simulink model "Main_simulation_optimised_BATTERYonly"  (R2017b)
settings: Solver=FixedStepDiscrete  StartTime=0  StopTime=20  RelTol=1e-3  EnableMultiTasking=on
PreLoadFcn:
  | Ts=2e-6;
undefined symbols (not defined in the file): DiscIntNeverNeededParam, Ion, Lithium, sigbuilder_block
libraries: powerlib x20, electricdrivelib x5, autolibshared x5, powerlib_meascontrol x3, sdolib x2, spsDrivesDcBusModel x1, spsDrivesPrivateModels x1, spsDrivesOutputSelector x1, spsDrivesSpeedControllerModel x1, simulink x1
(part 1 of 2)
Description:
  | Copyright 2008-2017 The MathWorks, Inc.
settings Model: SimulationMode=accelerator  ExtModeAutoUpdateStatusClock=off  Creator=MathWorks  LastModifiedBy=LENOVO
settings SolverCC: AlgebraicLoopSolver=LineSearch
settings DataIOCC: LimitDataPoints=on  SaveFormat=Array  SignalLoggingSaveFormat=ModelDataLogs  SaveOutput=off  SignalLogging=off  SaveTime=off  SignalLoggingName=sigsOut
settings OptimizationCC: ExpressionDepthLimit=2147483647  InitFltsAndDblsToZero=on  LifeSpan=inf
settings DebuggingCC: UnderspecifiedInitializationDetection=Classic  MergeDetectMultiDrivingBlocksExec=none  CheckExecutionContextPreStartOutputMsg=on  CheckExecutionContextRuntimeOutputMsg=on  SignalResolutionControl=TryResolveAllWithWarning  MultiTaskDSMMsg=warning  MultiTaskCondExecSysMsg=none  FcnCallInpInsideContextMsg=warning  StateNameClashWarn=warning  SFUnexpectedBacktrackingDiag=warning  SFNoUnconditionalDefaultTransitionDiag=warning  SFExecutionAtInitializationDiag=none
settings HardwareCC: ProdBitPerPointer=32  ProdBitPerSizeT=32  ProdBitPerPtrDiffT=32  ProdLargestAtomicFloat=None  ProdIntDivRoundTo=Undefined  ProdEndianess=Unspecified  ProdWordSize=32  ProdHWDeviceType=32-bit Generic  TargetUnknown=on
settings ModelReferenceCC: PropagateSignalLabelsOutOfModel=off
settings CodeAppCC: StateflowObjectComments=on
settings GRTTargetCC: TargetLangStandard=C89/C90 (ANSI)  GeneratePreprocessorConditionals=Disable all  CombineOutputUpdateFcns=off  GRTInterface=on
settings ConfigComp: CovMetricSettings=dw  CovHtmlReporting=on  CovSaveCumulativeToWorkspaceVar=on  CovSaveSingleToWorkspaceVar=on  CovExternalEMLEnable=off  CovSFcnEnable=off
settings SimscapeCC: SimscapeNormalizeSystem=off

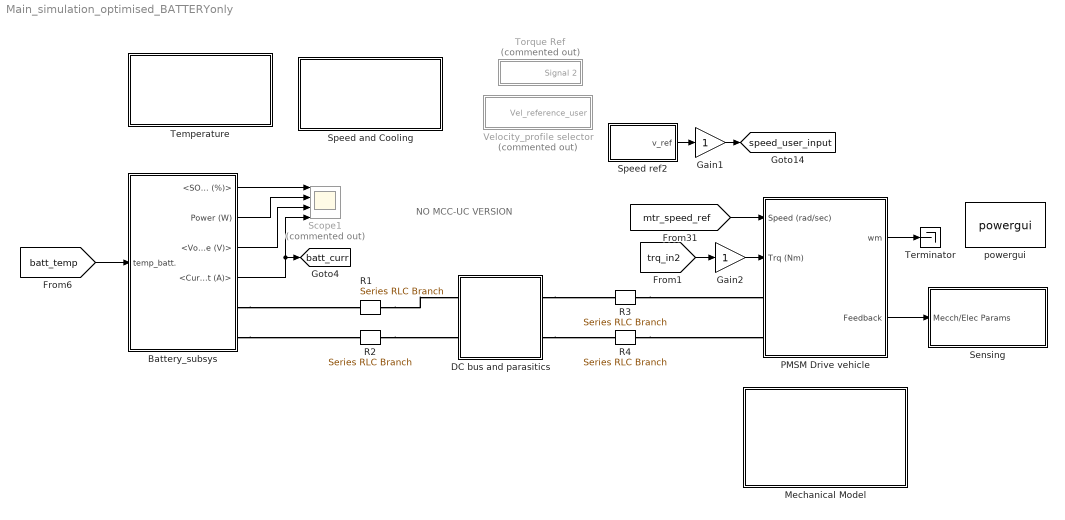
== system Main_simulation_optimised_BATTERYonly ==
  note: NO MCC-UC VERSION
  Battery_subsys : Subsystem
  DC bus and parasitics : Subsystem
  Gain1 : Gain
  Gain2 : Gain
  Mechanical Model : Subsystem
  PMSM Drive vehicle : Subsystem
  R{1..4} (4 alike) : powerlib/Elements/Series RLC Branch  LConnTagsString=__new0  RConnTagsString=__new0  BranchType=R  Resistance=0.02  Inductance=220e-6  SetiL0=off  InitialCurrent=0  Capacitance=447e-6  Setx0=off  InitialVoltage=0  Measurements=None
  Scope1 : Scope  Commented=on  NumInputPorts=4
  Sensing : Subsystem
  "Speed and Cooling " : Subsystem
  Speed ref2 : Subsystem  Tag=STV Subsys  LoadFcn=sigbuilder_block('load');  StartFcn=sigbuilder_block('start');  StopFcn=sigbuilder_block('stop');  ClipboardFcn=sigbuilder_block('clipboard');  mask(Sigbuilder block){tuvar=[0:10]}
      mask help: Simulink:masks:SigbuilderBlock_MD
      mask init:
      | if ~strcmp(get_param(bdroot(gcbh),'SimulationStatus'),'stopped') tuvar = sigbuilder_block('maskInit'); end
      settings: CopyFcn=sigbuilder_block('copy');  DeleteFcn=sigbuilder_block('delete');  ModelCloseFcn=sigbuilder_block('modelClose');  PreSaveFcn=sigbuilder_block('preSave');  PauseFcn=sigbuilder_block('pause');  ContinueFcn=sigbuilder_block('continue');  NameChangeFcn=sigbuilder_block('namechange');  OpenFcn=sigbuilder_block('open',[5.4 33 1141.2 514.8 ]);  CloseFcn=sigbuilder_block('close');
      mask Display: plot(0, 0, 100, 100,[2, 2, 32, 32, 2], [68, 8, 8, 68, 68],[32, 2], [38, 38], [32, 19, 2],[53, 60, 44], [32, 17, 17, 2],[16, 16, 31, 31]);txt = getActiveGroup(gcbh);text(2, 100, txt,'verticalAlignment', 'top');
  Temperature : Subsystem
  Terminator : Terminator
  Torque Ref : Subsystem  Tag=STV Subsys  Commented=on  LoadFcn=sigbuilder_block('load');  StartFcn=sigbuilder_block('start');  StopFcn=sigbuilder_block('stop');  ClipboardFcn=sigbuilder_block('clipboard');  mask(Sigbuilder block){tuvar=[0:10]}
      mask help: Simulink:masks:SigbuilderBlock_MD
      mask init:
      | if ~strcmp(get_param(bdroot(gcbh),'SimulationStatus'),'stopped') tuvar = sigbuilder_block('maskInit'); end
      settings: CopyFcn=sigbuilder_block('copy');  DeleteFcn=sigbuilder_block('delete');  ModelCloseFcn=sigbuilder_block('modelClose');  PreSaveFcn=sigbuilder_block('preSave');  PauseFcn=sigbuilder_block('pause');  ContinueFcn=sigbuilder_block('continue');  NameChangeFcn=sigbuilder_block('namechange');  OpenFcn=sigbuilder_block('open',[5.4 30 1141.2 522.6 ]);  CloseFcn=sigbuilder_block('close');
      mask Display: plot(0, 0, 100, 100,[2, 2, 32, 32, 2], [68, 8, 8, 68, 68],[32, 2], [38, 38], [32, 19, 2],[53, 60, 44], [32, 17, 17, 2],[16, 16, 31, 31]);txt = getActiveGroup(gcbh);text(2, 100, txt,'verticalAlignment', 'top');
  Velocity_profile selector : Subsystem  Commented=on
  powergui : powerlib/powergui  Priority=2  SimulationMode=Discrete  SampleTime=1e-6  frequency=60  Iterations=50  frequencyindice=0  Pbase=100e6  ErrMax=1e-4  UnitsV=kV  UnitsW=MW  buscounter=0  FunctionMessages=off  echomessages=off  EnableUseOfTLC=off  CurrentSourceSwitches=off  DisableSnubberDevices=off  DisableRonSwitches=off  DisableVfSwitches=off  DisplayEquations=off  SolverType=Tustin/Backward Euler (TBE)  Interpol=off  ExternalGateDelay=off  methode=off  Ts=0  x0status=blocks  SPID=off  SwTol=0  HookPort=off  RestoreLinks=warning  ResistiveCurrentMeasurement=off  Frange=[0:2:500]  Ylog=off  Xlog=on  ShowGrid=off  save=off  variable=ZData  structure=0  ZoomFFT=on  StartTime=0.0  cycles=1  DisplayStyle=1  fundamental=60  FreqAxis=off  MaxFrequency=1000  frequencyindicesteady=1  RmsSteady=1  display=off
  tag scope: batt_curr=global, speed_user_input=global
  wires:
  Speed ref2/1(v_ref) -> Gain1/1
  [trq_in2] -> Gain2/1
  Gain2/1 -> PMSM Drive vehicle/2(Trq (Nm))
  PMSM Drive vehicle/1(wm) -> Terminator/1
  PMSM Drive vehicle/2(Feedback) -> Sensing/1(Mecch/Elec Params)
  Battery_subsys/4(<Current (A)>) -> Scope1/4, [batt_curr]
  [batt_temp] -> Battery_subsys/1(temp_batt.)
  Battery_subsys/2(Power (W)) -> Scope1/2
  Battery_subsys/1(<SOC (%)>) -> Scope1/1
  Battery_subsys/3(<Voltage (V)>) -> Scope1/3
  [mtr_speed_ref] -> PMSM Drive vehicle/1(Speed (rad/sec))
  Gain1/1 -> [speed_user_input]
  connections:
  DC bus and parasitics/RConn1 -- R3/RConn1
  DC bus and parasitics/RConn2 -- R4/RConn1
  Battery_subsys/RConn1 -- R1/RConn1
  Battery_subsys/RConn2 -- R2/RConn1
  R1/LConn1 -- DC bus and parasitics/LConn1
  R2/LConn1 -- DC bus and parasitics/LConn2
  R3/LConn1 -- PMSM Drive vehicle/LConn1
  R4/LConn1 -- PMSM Drive vehicle/LConn2

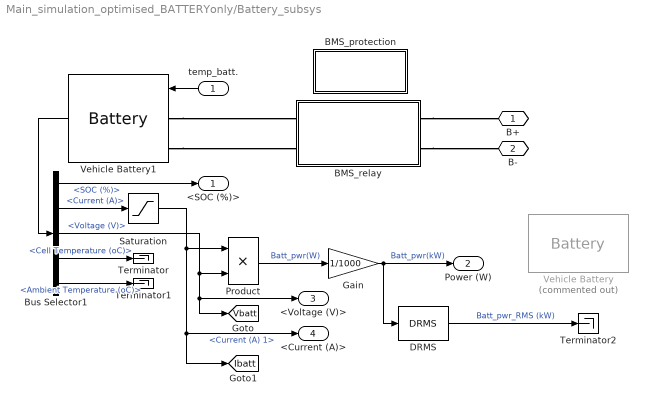
== system Main_simulation_optimised_BATTERYonly/Battery_subsys ==
  temp_batt. : Inport
  BMS_protection : Subsystem
  BMS_relay : Subsystem
  Bus Selector1 : BusSelector  OutputSignals=SOC (%),Current (A),Voltage (V),Cell Temperature (oC),Ambient Temperature (oC)
  DRMS : sdolib/RMS Blocks/DRMS  Ts=10e-6
      settings: SourceProductName=Simulink Design Optimization  SourceProductBaseCode=SO
  Gain : Gain  Gain=1/1000
  Product : Product
  Saturation : Saturate  UpperLimit=50  LowerLimit=-40
  Terminator : Terminator
  Terminator1 : Terminator
  Terminator2 : Terminator
  Vehicle Battery : electricdrivelib/Extra Sources/Battery  Commented=on  BatType=Lithium-Ion  ShowTempParam=off  ThermalPreset=no  ShowAgeParam=off  NomV=120  NomQ=66  SOC=80  Batt_Tr=30  PresetModel=off  MaxQ=66  MinV=90  FullV=130  Dis_rate=30  R=0.018182  Normal_OP=59.687  expZone="[129.6463      3.242609]"  current=[6.5 13 18 22 32.5 40]  Units=Time  Tci=20  NomT=50  T2=-15  MaxQ2=60*0.7  FullV2=117  Normal_OP2=120*0.9  expZone2="[120        50]"  Rca=0.06  ti=1000  Dp=0  Neq0=1  Tsim=1e6  Ta1=35  Qeol=60*0.85  Reol=0.013333*1.2  Char_age=[2.3478, 3]  Dis_age=[2.3478, 10]  N1=1500  N2=10500  N3=1000  N4=1400  Ta2=45  N5=950
  Vehicle Battery1 : electricdrivelib/Extra Sources/Battery  BatType=Lithium-Ion  ShowTempParam=on  ThermalPreset=no  ShowAgeParam=off  NomV=120  NomQ=66  SOC=100  Batt_Tr=0.1  PresetModel=off  MaxQ=66  MinV=90  FullV=130  Dis_rate=30  R=0.018182  Normal_OP=59.687  expZone="[129.6463      3.242609]"  current=[3.5 6.5 13 18 22 32.5 40]  Units=Time  Tci=20  NomT=50  T2=-15  MaxQ2=60*0.7  FullV2=117  Normal_OP2=120*0.9  expZone2="[120        50]"  Rca=0.5  ti=1  Dp=0  Neq0=1  Tsim=50e-6  Ta1=35  Qeol=60*0.85  Reol=0.013333*1.2  Char_age=[2.3478, 3]  Dis_age=[2.3478, 10]  N1=1500  N2=10500  N3=1000  N4=1400  Ta2=45  N5=950
  B+ : PMIOPort  Port=1  Side=Right
  B- : PMIOPort  Port=2  Side=Right
  <SOC (%)> : Outport
  Power (W) : Outport  Port=2
  <Voltage (V)> : Outport  Port=3
  <Current (A)> : Outport  Port=4
  tag scope: Ibatt=global, Vbatt=global
  wires:
  temp_batt./1 -> Vehicle Battery1/1
  Bus Selector1/2 -> Saturation/1  "<Current (A)>"
  Bus Selector1/1 -> <SOC (%)>/1  "<SOC (%)>"
  Product/1 -> Gain/1  "Batt_pwr(W)"
  Vehicle Battery1/1 -> Bus Selector1/1
  Bus Selector1/3 -> <Voltage (V)>/1, [Vbatt], Product/2  "<Voltage (V)>"
  Gain/1 -> DRMS/1, Power (W)/1  "Batt_pwr(kW)"
  Saturation/1 -> <Current (A)>/1, [Ibatt], Product/1  "<Current (A) 1>"
  Bus Selector1/4 -> Terminator/1  "<Cell Temperature (oC)>"
  Bus Selector1/5 -> Terminator1/1  "<Ambient Temperature (oC)>"
  DRMS/1 -> Terminator2/1  "Batt_pwr_RMS (kW)"
  connections:
  Vehicle Battery1/LConn1 -- BMS_relay/LConn1
  Vehicle Battery1/LConn2 -- BMS_relay/LConn2
  BMS_relay/RConn1 -- B+/RConn1
  BMS_relay/RConn2 -- B-/RConn1

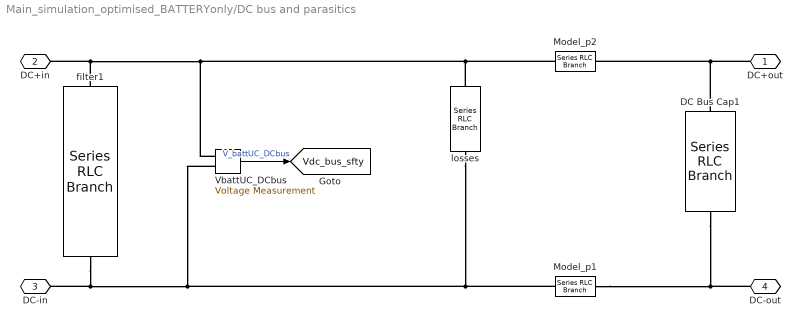
== system Main_simulation_optimised_BATTERYonly/DC bus and parasitics ==
  DC Bus Cap1 : powerlib/Elements/Series RLC Branch  LConnTagsString=__new0  RConnTagsString=__new0  BranchType=RC  Resistance=1e-2  Inductance=1e-3  SetiL0=off  InitialCurrent=0  Capacitance=400e-6  Setx0=off  InitialVoltage=0  Measurements=None
  Model_p1 : powerlib/Elements/Series RLC Branch  LConnTagsString=__new0  RConnTagsString=__new0  BranchType=RL  Resistance=0.01  Inductance=20e-6  SetiL0=off  InitialCurrent=0  Capacitance=0  Setx0=off  InitialVoltage=0  Measurements=None
  Model_p2 : powerlib/Elements/Series RLC Branch  LConnTagsString=__new0  RConnTagsString=__new0  BranchType=RL  Resistance=0.01  Inductance=20e-6  SetiL0=off  InitialCurrent=0  Capacitance=0  Setx0=off  InitialVoltage=0  Measurements=None
  VbattUC_DCbus : powerlib/Measurements/Voltage Measurement  PhasorSimulation=off  OutputType=Complex  PSBequivalent=0
  filter1 : powerlib/Elements/Series RLC Branch  LConnTagsString=__new0  RConnTagsString=__new0  BranchType=RC  Resistance=1e-3  Inductance=1e-3  SetiL0=off  InitialCurrent=0  Capacitance=1e-6  Setx0=off  InitialVoltage=0  Measurements=None
  losses : powerlib/Elements/Series RLC Branch  LConnTagsString=__new0  RConnTagsString=__new0  BranchType=R  Resistance=100e3  Inductance=1e-3  SetiL0=off  InitialCurrent=0  Capacitance=1e-6  Setx0=off  InitialVoltage=0  Measurements=None
  DC+out : PMIOPort  Port=1  Side=Right
  DC+in : PMIOPort  Port=2  Side=Left
  DC-in : PMIOPort  Port=3  Side=Left
  DC-out : PMIOPort  Port=4  Side=Right
  tag scope: Vdc_bus_sfty=global
  wires:
  VbattUC_DCbus/1 -> [Vdc_bus_sfty]  "V_battUC_DCbus"
  connections:
  DC-out/RConn1 -- Model_p1/LConn1 -- DC Bus Cap1/RConn1
  Model_p2/LConn1 -- DC+out/RConn1 -- DC Bus Cap1/LConn1
  filter1/RConn1 -- Model_p1/RConn1 -- losses/RConn1 -- VbattUC_DCbus/LConn2 -- DC-in/RConn1
  filter1/LConn1 -- Model_p2/RConn1 -- losses/LConn1 -- VbattUC_DCbus/LConn1 -- DC+in/RConn1

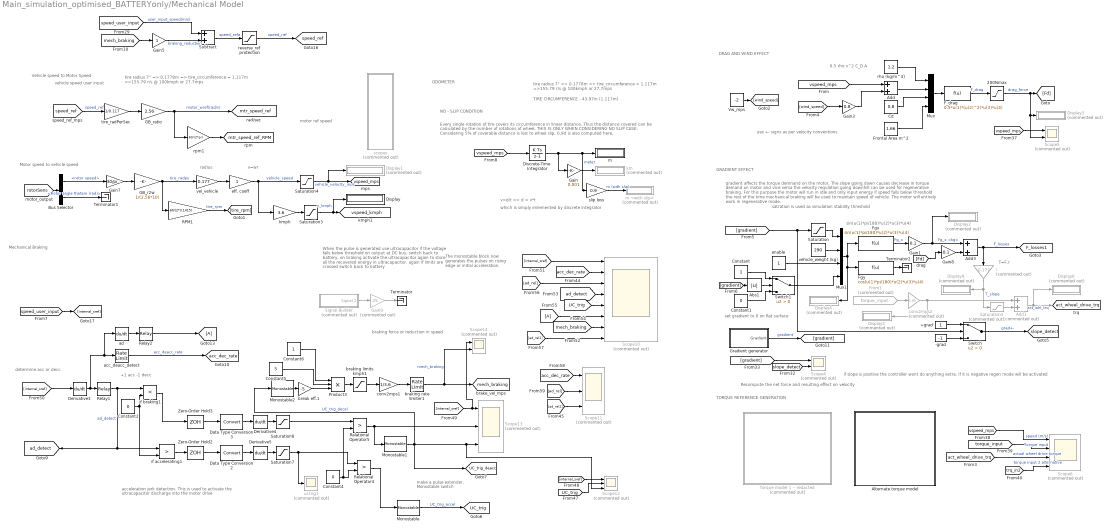
== system Main_simulation_optimised_BATTERYonly/Mechanical Model ==
  note: which is simply imlemented by discrete integrator
  note: v=d/t => d = v*t
  note: Every single rotation of tire covers its circumference in linear distance. Thus the distance covered
      | can be calculated by the number of rotations of wheel. THIS IS ONLY WHEN CONSIDERING
      | NO SLIP CASE. Considering 5% of coverable distance is lost to wheel slip, 0.9d is also computed here.
  note: TIRE CIRCUMFERENCE - 43.97in (1.117m)
  note: NO - SLIP CONDITION
  note: ODOMETER
  note: sin(u(1)*pi/180)*u(2)*u(3)*u(4)
  note: set gradient to 0 on flat surface
  note: Recompute the net force and resulting effect on velocity
  note: Vehicle speed to Motor Speed
  note: motor ref speed
  note: tire radius 7" => 0.1778m => tire_circumference = 1.117m
      | =>155.79 r/s @ 100kmph or 27.7mps
  note: vehicle speed
      | user input
  note: v=wr
  note: Motor speed to vehicle speed
  note: radius
  note: T=F.r
  note: use +- signs as per velocity conventions
  note: satration is used as simulation stability threshold
  note: gradient affects the torque demnand on the motor. The slope going down causes decrease in torque demand on motor and vice versa
      |
      | the velocity regulation going downhill can be used for regenerative braking. For this purpose the motor will run in idle and only input energy if speed falls below threshold
      | the rest of the time mechanical braking will be used to maintain speed of vehicle. The motor will entirely work in regenerative mode.
  note: if slope is positive the controller wont do anything extra. If it is negative regen mode will be activated
  note: 0.5 rho v^2 C_D A
  note: GRADIENT EFFECT
  note: DRAG AND WIND EFFECT
  note: TORQUE REFERENCE GENERATION
  note: make a pulse extender.
      | Monostable switch
  note: acceleration jerk detection. This is used to activate the ultracapacitor discharge into the motor drive
  note: When the pulse is generated use ultracapacitor
      | if the voltage falls below threshold on output
      | at DC bus, switch back to battery.
      |
      | on braking activate the ultracapacitor again to store all
      | the recovered energy in ultracapacitor. again if limits are
      | crossed switch back to battery
  note: The monostable block
      | now generates the
      | pulses on rising edge or
      | initial acceleration.
  note: Mechanical Braking
  note: braking force or reduction in speed
  note: determine acc or decc
  note: +1 acc
      |  -1 decc
  note: tire radius 7" => 0.1778m => tire_circumference = 1.117m
      | =>155.79 r/s @ 100kmph or 27.7mps
  +grad : Constant
  -grad : Constant  Value=-1
  200Nmax : Saturate  UpperLimit=200  LowerLimit=0
  Abs1 : Abs
  Add : Sum
  Add1 : Sum  Commented=on
  Add3 : Sum
  Alternate torque model : Subsystem
  Bus Selector : BusSelector  OutputSignals=rotor speed,Rotor angle thetam (rad)
  Cd : Constant  Value=0.8
  Constant : Constant
  Constant1 : Constant  Value=0
  Constant2 : Constant  Value=0
  Constant4 : Constant  Value=0
  Constant5 : Constant  Value=5
  Constant6 : Constant
  Data Type Conversion2 : DataTypeConversion
  Data Type Conversion3 : DataTypeConversion
  Derivative3 : Derivative
  Derivative4 : Derivative
  Derivative5 : Derivative
  Discrete-Time Integrator : DiscreteIntegrator  InitialConditionSetting=State (most efficient)  SampleTime=-1  ICPrevOutput=DiscIntNeverNeededParam  ICPrevScaledInput=DiscIntNeverNeededParam
  Display : Display
  Display{1..6,9} (7 alike) : Display  Commented=on
  F_drag : Fcn  Expr=0.5*u(1)*(u(2)^2)*u(3)*u(4)
  Fgx : Fcn  Expr=sin(u(1)*pi/180)*u(2)*u(3)*u(4)
  Fgy : Fcn  Expr=cos(u(1)*pi/180)*u(2)*u(3)*u(4)
  From1 : From  Commented=on  GotoTag=torque_input  TagVisibility=global
  Frontal Area m^2 : Constant  Value=1.66
  GB_r2w : Gain  Gain=1/(2.56*10)
  GB_ratio : Gain  Gain=2.56
  Gain : Gain  Gain=0.001
  Gain1 : Gain  Gain=0.1
  Gain3 : Gain  Gain=0.8
  Gain5 : Gain
  Gain7 : Gain  Gain=30/pi  SaturateOnIntegerOverflow=on  OutDataTypeStr=Inherit: Same as input  ParamDataTypeStr=Inherit: Same as input
  Gain8 : Gain  Gain=0.1
  Gain9 : Gain  Commented=on  Gain=25
  Gradient generator : Subsystem  Tag=STV Subsys  LoadFcn=sigbuilder_block('load');  StartFcn=sigbuilder_block('start');  StopFcn=sigbuilder_block('stop');  ClipboardFcn=sigbuilder_block('clipboard');  mask(Sigbuilder block){tuvar=[0:10]}
      mask help: Simulink:masks:SigbuilderBlock_MD
      mask init:
      | if ~strcmp(get_param(bdroot(gcbh),'SimulationStatus'),'stopped') tuvar = sigbuilder_block('maskInit'); end
      settings: CopyFcn=sigbuilder_block('copy');  DeleteFcn=sigbuilder_block('delete');  ModelCloseFcn=sigbuilder_block('modelClose');  PreSaveFcn=sigbuilder_block('preSave');  PauseFcn=sigbuilder_block('pause');  ContinueFcn=sigbuilder_block('continue');  NameChangeFcn=sigbuilder_block('namechange');  OpenFcn=sigbuilder_block('open',[0 30 1152 561.6 ]);  CloseFcn=sigbuilder_block('close');
      mask Display: plot(0, 0, 100, 100,[2, 2, 32, 32, 2], [68, 8, 8, 68, 68],[32, 2], [38, 38], [32, 19, 2],[53, 60, 44], [32, 17, 17, 2],[16, 16, 31, 31]);txt = getActiveGroup(gcbh);text(2, 100, txt,'verticalAlignment', 'top');
  Monostable : powerlib_meascontrol/Logic/Monostable  EdgeDetect=Rising  PulseDuration=0.4  ic=0  Ts=0
      settings: SourceProductName=Simscape Power Systems  SourceProductBaseCode=PS
  Monostable1 : powerlib_meascontrol/Logic/Monostable  EdgeDetect=Rising  PulseDuration=0.15  ic=0  Ts=0
      settings: SourceProductName=Simscape Power Systems  SourceProductBaseCode=PS
  Monostable2 : powerlib_meascontrol/Logic/Monostable  EdgeDetect=Rising  PulseDuration=0.45  ic=0  Ts=0
      settings: SourceProductName=Simscape Power Systems  SourceProductBaseCode=PS
  Mux : Mux
  Mux1 : Mux
  Product3 : Product  Inputs=3
  RPM1 : Gain  Gain=60/(2*3.1415)
  Relational Operator4 : RelationalOperator  Operator=>  OutDataTypeStr=boolean  RndMeth=Simplest
  Relational Operator5 : RelationalOperator  Operator=>  OutDataTypeStr=boolean  RndMeth=Simplest
  Relay1 : Relay  OffOutputValue=-1
  Relay2 : Relay  OffOutputValue=-1
  Saturation : Saturate  UpperLimit=10  LowerLimit=-10
  Saturation3 : Saturate  UpperLimit=108  LowerLimit=0
  Saturation4 : Saturate  UpperLimit=30  LowerLimit=0
  Saturation5 : Saturate  Commented=on  UpperLimit=25  LowerLimit=-25
  Saturation7 : Saturate  UpperLimit=10  LowerLimit=-10
  Saturation8 : Saturate  UpperLimit=10  LowerLimit=-10
  Scope10 : Scope  Commented=on  NumInputPorts=8
  Scope11 : Scope  Commented=on  NumInputPorts=3
  Scope12 : Scope  Commented=on  NumInputPorts=3
  Scope13 : Scope  Commented=on  NumInputPorts=3
  Scope14 : Scope  Commented=on  NumInputPorts=2
  Scope4 : Scope  Commented=on  NumInputPorts=2
  Scope5 : Scope  Commented=on  NumInputPorts=2
  Scope6 : Scope  Commented=on  NumInputPorts=4
  Signal Builder : Subsystem  Tag=STV Subsys  Commented=on  LoadFcn=sigbuilder_block('load');  StartFcn=sigbuilder_block('start');  StopFcn=sigbuilder_block('stop');  ClipboardFcn=sigbuilder_block('clipboard');  mask(Sigbuilder block){tuvar=[0:10]}
      mask help: Simulink:masks:SigbuilderBlock_MD
      mask init:
      | if ~strcmp(get_param(bdroot(gcbh),'SimulationStatus'),'stopped') tuvar = sigbuilder_block('maskInit'); end
      settings: CopyFcn=sigbuilder_block('copy');  DeleteFcn=sigbuilder_block('delete');  ModelCloseFcn=sigbuilder_block('modelClose');  PreSaveFcn=sigbuilder_block('preSave');  PauseFcn=sigbuilder_block('pause');  ContinueFcn=sigbuilder_block('continue');  NameChangeFcn=sigbuilder_block('namechange');  OpenFcn=sigbuilder_block('open',[5.4 30 1141.2 522.6 ]);  CloseFcn=sigbuilder_block('close');
      mask Display: plot(0, 0, 100, 100,[2, 2, 32, 32, 2], [68, 8, 8, 68, 68],[32, 2], [38, 38], [32, 19, 2],[53, 60, 44], [32, 17, 17, 2],[16, 16, 31, 31]);txt = getActiveGroup(gcbh);text(2, 100, txt,'verticalAlignment', 'top');
  Subtract : Sum
  Switch : Switch  Criteria=u2 > Threshold
  Switch1 : Switch  Criteria=u2 > Threshold
  Terminator : Terminator
  Terminator1 : Terminator
  Terminator2 : Terminator
  "Torque model 1 -- redacted" : Subsystem  Commented=on
  Vw_mps : Constant  Value=-2
  Zero-Order Hold2 : ZeroOrderHold  SampleTime=-1
  Zero-Order Hold3 : ZeroOrderHold  SampleTime=-1
  acc_deacc_detect : RateLimiter  RisingSlewLimit=1000  FallingSlewLimit=-10e5  SampleTimeMode=inherited
  ad : Derivative
  braking limits kmph1 : Saturate  UpperLimit=0  LowerLimit=-40
  braking rate limiter1 : RateLimiter  RisingSlewLimit=10  FallingSlewLimit=-100  SampleTimeMode=inherited
  break eff.1 : Gain  Gain=-5
  conv2mps1 : Gain  Gain=1/3.6
  conv2mps2 : Gain  Commented=on  Gain=1.65
  eff. coeff : Gain
  enable : Constant
  if accelerating1 : RelationalOperator  Operator=>  OutDataTypeStr=boolean  RndMeth=Simplest
  if braking1 : RelationalOperator  Operator=<  OutDataTypeStr=boolean  RndMeth=Simplest
  km : Display  Commented=on
  kmph : Gain  Gain=3.6
  m : Display
  m <with slip> : Display  Commented=on
  r : Gain  Commented=on  Gain=0.177
  reverse_ref protection : Saturate  UpperLimit=45  LowerLimit=0
  rho (kg/m^3) : Constant  Value=1.2
  rpm1 : Gain  Gain=60/(2*pi)
  scopes : Subsystem  Commented=on
  slip loss : Gain  Gain=0.9
  tire_radPerSec : Gain  Gain=1/0.117
  uctrig1 : Scope  Commented=on
  vehicle_weight (kg) : Constant  Value=290
  vel_vehicle : Gain  Gain=0.177
  tag scope: F_losses1=global, UC_trig=global, UC_trig_deacc=global, acc_dec_rate=global, act_wheel_drive_trq=global, ad_detect=global, mech_braking=global, mtr_speed_ref=global, mtr_speed_ref_RPM=global, slope_detect=global, speed_ref=global, vspeed_kmph=global, vspeed_mps=global
  wires:
  GB_ratio/1 -> rpm1/1, [mtr_speed_ref]  "motor_wref(rad/s)"
  Bus Selector/1 -> Gain7/1  "<rotor speed>"
  Bus Selector/2 -> Terminator1/1  "<Rotor angle thetam (rad)>"
  vel_vehicle/1 -> eff. coeff/1
  RPM1/1 -> [tire_rpm]  "tire_rpm"
  kmph/1 -> Saturation3/1
  Gain3/1 -> Add/2
  Add3/1 -> [F_losses1], r/1  "F_losses"
  Saturation4/1 -> Display1/1, [vspeed_mps]  "vehicle_velocity_mps"
  GB_r2w/1 -> RPM1/1, vel_vehicle/1  "tire_radps"
  [Fd] -> Gain8/1
  [speed_ref] -> tire_radPerSec/1  "speed_ref"
  [rotorSens] -> Bus Selector/1
  eff. coeff/1 -> Saturation4/1, kmph/1  "vehicle_speed"
  Vw_mps/1 -> [wind_speed]
  r/1 -> Display9/1, Saturation5/1  "T_slope"
  F_drag/1 -> 200Nmax/1  "F_drag"
  tire_radPerSec/1 -> GB_ratio/1
  rho (kg/m^3)/1 -> Mux/1
  rpm1/1 -> [mtr_speed_ref_RPM]
  Saturation3/1 -> [vspeed_kmph], Display/1  "v_kmph"
  Mux1/1 -> Fgx/1, Display4/1, Fgy/1
  Gradient generator/1(Gradient) -> [gradient]  "gradient"
  Frontal Area m^2/1 -> Mux/4
  Fgx/1 -> Gain1/1  "Fg_x"
  -grad/1 -> Switch/3
  [vspeed_mps] -> Add/1
  Cd/1 -> Mux/3
  From1/1 -> conv2mps2/1
  Add/1 -> Mux/2
  Add1/1 -> Display6/1, [act_wheel_drive_trq]  "act_whl_trq"
  Mux/1 -> F_drag/1
  Fgy/1 -> Terminator2/1
  [wind_speed] -> Gain3/1
  Switch/1 -> [slope_detect]  "grad+-"
  [gradient] -> Switch/2, Saturation/1
  +grad/1 -> Switch/1
  vehicle_weight (kg)/1 -> Mux1/2
  Gain7/1 -> GB_r2w/1
  [speed_user_input] -> Subtract/1  "user_input_speed(m/s)"
  Subtract/1 -> reverse_ref protection/1  "speed_refa"
  [vspeed_mps] -> Scope5/1
  [trq_in2] -> Scope6/4  "torque input 2 alternative"
  [act_wheel_drive_trq] -> Scope6/3  "actual wheel drive torque"
  [vspeed_mps] -> Scope6/1  "speed (m/s)"
  Gain8/1 -> Add3/2
  200Nmax/1 -> Scope5/2, Display3/1, [Fd]  "drag_force"
  [slope_detect] -> Scope4/2
  Gain5/1 -> Subtract/2  "braking_reduction"
  conv2mps1/1 -> braking rate limiter1/1
  [internal_sref] -> Derivative3/1
  [mech_braking] -> Gain5/1
  [gradient] -> Scope4/1
  [torque_input] -> Scope6/2  "Torque input"
  ad/1 -> Relay2/1
  Derivative5/1 -> Saturation7/1
  Relational Operator4/1 -> Monostable/1
  Constant2/1 -> if accelerating1/2, if braking1/2
  [ad_detect] -> Scope10/4
  [mech_braking] -> Scope10/7
  Data Type Conversion3/1 -> Derivative4/1
  Monostable1/1 -> Scope12/3, Scope13/3, [UC_trig_deacc], Monostable2/1  "UC_trig_decel"
  [ad_rel] -> Scope10/3
  [UC_trig] -> Scope12/2
  Saturation7/1 -> uctrig1/1, Relational Operator4/1
  [internal_sref] -> Scope12/1
  acc_deacc_detect/1 -> [acc_dec_rate]  "acc_deacc_rate"
  braking rate limiter1/1 -> Scope14/2, [mech_braking]  "mech_braking"
  Data Type Conversion2/1 -> Derivative5/1
  [ad_rel] -> Scope11/2
  Relational Operator5/1 -> Monostable1/1, Scope13/2
  [ad_rel2] -> Scope10/8
  Zero-Order Hold2/1 -> Data Type Conversion2/1
  [ad_rel2] -> Scope11/3
  braking limits kmph1/1 -> conv2mps1/1
  Relay2/1 -> [A]
  Constant5/1 -> Product3/2
  Monostable2/1 -> break eff.1/1
  Zero-Order Hold3/1 -> Data Type Conversion3/1
  [acc_dec_rate] -> Scope11/1
  Gain9/1 -> Terminator/1
  [UC_trig] -> Scope10/5
  Derivative4/1 -> Saturation8/1
  Monostable/1 -> [UC_trig]  "UC_trig_accel"
  [internal_sref] -> Scope14/1, Scope13/1
  [speed_user_input] -> [internal_sref]
  if accelerating1/1 -> Zero-Order Hold2/1
  Constant4/1 -> Relational Operator5/2, Relational Operator4/2
  Saturation8/1 -> Relational Operator5/1
  Constant6/1 -> Product3/1
  Signal Builder/1(Signal 2) -> Gain9/1
  break eff.1/1 -> Product3/3
  if braking1/1 -> Zero-Order Hold3/1
  [A] -> Scope10/6
  Derivative3/1 -> ad/1, acc_deacc_detect/1, Relay1/1
  Product3/1 -> braking limits kmph1/1
  Relay1/1 -> [ad_detect], if accelerating1/1, if braking1/1  "ad_detect"
  [internal_sref] -> Scope10/1
  [acc_dec_rate] -> Scope10/2
  Saturation5/1 -> Add1/2
  conv2mps2/1 -> Display5/1, Add1/1
  Gain1/1 -> Display2/1, Add3/1  "Fg_x <kg>"
  enable/1 -> Mux1/3
  [gradient] -> Abs1/1
  Abs1/1 -> Switch1/2
  Constant/1 -> Switch1/1
  Constant1/1 -> Switch1/3
  Switch1/1 -> Mux1/4
  Saturation/1 -> Mux1/1
  reverse_ref protection/1 -> [speed_ref]  "speed_ref"
  [vspeed_mps] -> Discrete-Time Integrator/1
  Discrete-Time Integrator/1 -> Gain/1, slip loss/1, m/1  "meter"
  Gain/1 -> km/1
  slip loss/1 -> m <with slip>/1  "m (with slip)"

== system Main_simulation_optimised_BATTERYonly/PMSM Drive vehicle ==
  Speed (rad/sec) : Inport
  Trq (Nm) : Inport  Port=2
  Bus Creator : BusCreator  Inputs=3
  Bus Selector : BusSelector  OutputSignals=V bus (V)
  DC_bus overvoltage protection : Subsystem  Commented=on
  PM Synchronous Motor Drive : Subsystem  DialogController=POWERSYS.PowerSysDialog  LoadFcn=|  mask(PM Synchronous Motor Drive){Rs=0.2, Lls=8.5e-3, Lms=8.5e-3, MachineConstant=Flux linkage established by magnets (V.s), FluxCst=0.175, VoltageCst=126.966, TorqueCst=1.05, ia=0, ib=0, J=0.089, Friction=0.005, p=4, wm=0, thetam=0, Rsnb_rec=10e3, Csnb_rec=20e-9, Ron_rec=1e-3, Vf_rec=1.3, cap_bus=200e-6, Rbrake=8, fbrake=4000, activationVoltage=190, shutdownVoltage=175, sourceFrequency=60, deviceType=IGBT / Diodes, Ron_inv=1e-3, Vf_inv=0.8, Vfd_inv=0.8, Tf=1e-6, Tt=2e-6, Tf_GTO=0, Tt_GTO=0, Rsnb_inv=5000, Csnb_inv=inf, regulationType=Speed regulation, Acc=1000, Dec=-1000, kp_sc=5, ki_sc=100, fc_sc=100, Tsc=7*20e-6, Tmin=-17.8, Tmax=17.8, modulationType=Hysteresis, h=0.1, kp_Id=200, ki_Id=1000, kp_Iq=200, ki_Iq=1000, fc_bus=50, car_freq=20000, freq_max=20e3, Tvect=20e-6, baseSampleTime=2e-06, outputBusMode=Multiple output buses, busLabels=off, MechanicalLoad=Torque Tm, modelDetailLevel=Detailed, driveType=AC6, AverageValue=off}
      | if ~isempty(get_param(gcb,'UserData')) 
      |       UserDataToSimulinkMask(gcbh,get_param(gcb,'driveType'));  
      |       set_param(gcb, 'UserData',[]);
      |       set_param(gcb,'UserDataPersistent','off');
      | end 
      | if strcmp(get_param(gcb,'AverageValue'),'on')
      |     set_param(gcb,'modelDetailLevel','Average');
      | end
      mask prompts: Rs "Resistance (ohm):"; Lls "D-axis inductance (H):"; Lms "Q-axis inductance (H):"; MachineConstant "Specify:"; ia "Phase A (A):"; ib "Phase B (A):"; J "Inertia (kg.m^2):"; Friction "Friction factor (N.m.s):"; p "Pole pairs:"; wm "Speed (rad/s):"; thetam "Angle (deg):"; Rsnb_rec "Resistance (ohm):"; Csnb_rec "Capacitance (F):"; Ron_rec "On-state resistance (ohm):"; Vf_rec "Forward voltage (V):"; cap_bus "Capacitance (F):"; Rbrake "Resistance (ohm):"; fbrake "Chopper frequency (Hz):"; activationVoltage "Activation voltage (V):"; shutdownVoltage "Shutdown voltage (V):"; sourceFrequency "Source frequency (Hz):"; deviceType "Device type:"; Ron_inv "On-state resistance (ohm):"; Vf_inv "Main device:"; Vfd_inv "Diode:"; Tf "Fall time (s):"; Tt "Tail time (s):"; Tf_GTO "Fall time (s):"; Tt_GTO "Tail time (s):"; Rsnb_inv "Resistance (ohm):"; Csnb_inv "Capacitance (F):"; regulationType "Regulation type:"; Acc "Acceleration:"; Dec "Deceleration:"; kp_sc "Proportional gain:"; ki_sc "Integral gain:"; fc_sc "Speed cutoff frequency (Hz):"; Tsc "Speed controller sampling time (s):"; Tmin "Negative:"; Tmax "Positive:"; modulationType "Modulation type:"; h "Current controller hysteresis bandwidth (A):"; kp_Id "Proportional gain:"; ki_Id "Integral gain:"; kp_Iq "Proportional gain:"; ki_Iq "Integral gain:"; fc_bus "DC bus voltage sensor cutoff frequency (Hz):"; car_freq "SVM switching frequency (Hz):"; freq_max "Maximum  switching frequency (Hz):"; Tvect "Controller sampling time (s):"; baseSampleTime "Base sample time:"; outputBusMode "Output bus mode:"; busLabels "Use bus labels"; MechanicalLoad "Mechanical input:"; modelDetailLevel "Model detail level:"; driveType "Drive type:"; AverageValue "Average value model"
      mask help: Implements a classical vector control drive for permanent synchronous motors.
      mask init:
      | [X1,X1m,X2,X2m,X3,X4,Y1,Y1m,Y2,Y2m,Y3,Y4,color1,color2,INp,OUTp,machineType,baseSampleTime] = spsDrivesMaskInit(gcb,driveType,AverageValue);
      settings: OpenFcn=sps_rtmsupport('OpenFcn',gcbh)
      mask Help: helpview(psbhelp)
      mask TypeOptions MachineConstant: Flux linkage established by magnets (V.s) | Voltage Constant (V_peak L-L / krpm) | Torque Constant (N.m / A_peak)
      mask Callback MachineConstant:
      | block = gcb;
      | MC = get_param(block,'MachineConstant');
      | set_param([block,'/','Permanent Magnet Synchronous Machine'],'MachineConstant',MC);
      | set_param([block,'/','VECT'],'MachineConstant',MC);
      | switch MC
      |     case 'Flux linkage established by magnets (V.s)'
      |         set_param([block,'/','Permanent Magnet Synchronous Machine'],'Flux',get_param(block,'FluxCst'))
      |     case 'Voltage Constant (V_peak L-L / krpm)'
      |         set_param([block,'/','Permanent Magnet Synchronous Machine'],'VoltageCst',get_param(block,'VoltageCst'))
      |     case 'Torque Constant (N.m / A_peak)'
      |         set_param([block,'/','Permanent Magnet Synchronous Machine'],'TorqueCst',get_param(block,'TorqueCst'))
      | end
      mask Callback FluxCst:
      | block = gcb;
      | MC = get_param(block,'MachineConstant');
      | set_param([block,'/','Permanent Magnet Synchronous Machine'],'MachineConstant',MC);
      | set_param([block,'/','VECT'],'MachineConstant',MC);
      | switch MC
      |     case 'Flux linkage established by magnets (V.s)'
      |         set_param([block,'/','Permanent Magnet Synchronous Machine'],'Flux',get_param(block,'FluxCst'))
      |     case 'Voltage Constant (V_peak L-L / krpm)'
      |         set_param([block,'/','Permanent Magnet Synchronous Machine'],'VoltageCst',get_param(block,'VoltageCst'))
      |     case 'Torque Constant (N.m / A_peak)'
      |         set_param([block,'/','Permanent Magnet Synchronous Machine'],'TorqueCst',get_param(block,'TorqueCst'))
      | end
      mask Callback VoltageCst:
      | block = gcb;
      | MC = get_param(block,'MachineConstant');
      | set_param([block,'/','Permanent Magnet Synchronous Machine'],'MachineConstant',MC);
      | set_param([block,'/','VECT'],'MachineConstant',MC);
      | switch MC
      |     case 'Flux linkage established by magnets (V.s)'
      |         set_param([block,'/','Permanent Magnet Synchronous Machine'],'Flux',get_param(block,'FluxCst'))
      |     case 'Voltage Constant (V_peak L-L / krpm)'
      |         set_param([block,'/','Permanent Magnet Synchronous Machine'],'VoltageCst',get_param(block,'VoltageCst'))
      |     case 'Torque Constant (N.m / A_peak)'
      |         set_param([block,'/','Permanent Magnet Synchronous Machine'],'TorqueCst',get_param(block,'TorqueCst'))
      | end
      mask Callback TorqueCst:
      | block = gcb;
      | MC = get_param(block,'MachineConstant');
      | set_param([block,'/','Permanent Magnet Synchronous Machine'],'MachineConstant',MC);
      | set_param([block,'/','VECT'],'MachineConstant',MC);
      | switch MC
      |     case 'Flux linkage established by magnets (V.s)'
      |         set_param([block,'/','Permanent Magnet Synchronous Machine'],'Flux',get_param(block,'FluxCst'))
      |     case 'Voltage Constant (V_peak L-L / krpm)'
      |         set_param([block,'/','Permanent Magnet Synchronous Machine'],'VoltageCst',get_param(block,'VoltageCst'))
      |     case 'Torque Constant (N.m / A_peak)'
      |         set_param([block,'/','Permanent Magnet Synchronous Machine'],'TorqueCst',get_param(block,'TorqueCst'))
      | end
      mask TypeOptions deviceType: GTO / Diodes | MOSFET / Diodes | IGBT / Diodes
      mask Callback deviceType: set_param([gcb,'/Three-phase Inverter'],'Device',get_param(gcb,'deviceType'));
      mask TypeOptions regulationType: Speed regulation | Torque regulation
      mask Callback regulationType: set_param([gcb '/Speed Controller'],'SwK',get_param(gcb,'regulationType'));
      mask TypeOptions modulationType: Hysteresis | SVM
      mask TypeOptions outputBusMode: Multiple output buses | Single output bus
      mask TypeOptions MechanicalLoad: Torque Tm | Speed w | Mechanical rotational port
      mask TypeOptions modelDetailLevel: Detailed | Average
      mask Callback modelDetailLevel:
      | if strcmp(get_param(gcb,'modelDetailLevel'),'Average')
      |    set_param(gcb,'AverageValue','on');
      | else
      |    set_param(gcb,'AverageValue','off');
      | end
      mask TypeOptions driveType: AC6
      mask DialogControl Container7 Prompt: Permanent Magnet Synchronous Machine
      mask DialogControl Container22 Prompt: Electrical parameters
      mask DialogControl Container27 Prompt: Equivalent circuit parameters
      mask DialogControl Container21 Prompt: Flux constant
      mask DialogControl Container34 Prompt: Initial currents
      mask DialogControl Container23 Prompt: Mechanical parameters
      mask DialogControl Container36 Prompt: Initial  values
      mask DialogControl Container10 Prompt: Converters and DC bus
      mask DialogControl Container28 Prompt: Rectifier
      mask DialogControl Container26 Prompt: Snubbers
      mask DialogControl Container29 Prompt: Diodes
      mask DialogControl Container30 Prompt: DC bus
      mask DialogControl Container31 Prompt: Braking chopper
      mask DialogControl Container32 Prompt: Inverter
      mask DialogControl Container37 Prompt: Switches
      mask DialogControl Forwardvoltages Prompt: Forward voltages (V)
      mask DialogControl Turnoff Prompt: Turn-off characteristics
      mask DialogControl InvSnubbers Prompt: Snubbers
      mask DialogControl Container12 Prompt: Controller
      mask DialogControl Control5 Prompt: Schematic
      mask DialogControl Control5 Callback:
      | openfig('ac6.fig','invisible');
      | movegui(gcf,'northwest');
      | set(gcf,'Visible','on');
      mask DialogControl Container33 Prompt: Speed controller
      mask DialogControl Speedramp Prompt: Speed ramps (rpm/s)
      mask DialogControl PIregulator Prompt: PI regulator
      mask DialogControl Container43 Prompt: Torque output limits (N.m)
      mask DialogControl Container35 Prompt: Vector control
      mask DialogControl d_axiscurrentregulator Prompt: d-axis current regulator
      mask DialogControl q_axiscurrentregulator Prompt: q-axis current regulator
      mask DialogControl Container47 Prompt: Parameters file options
      mask DialogControl Control3 Prompt: Load
      mask DialogControl Control3 Callback: loadValues(gcb,get_param(gcb,'driveType'));
      mask DialogControl Control4 Prompt: Save
      mask DialogControl Control4 Callback: saveValues(gcb,get_param(gcb,'driveType'));
      mask Display:
      | patch([X1 X1m],[Y1 Y1m],color1);
      | patch(X3,Y3,color2);
      | plot([X1 X1m X2 X2m X3 X4],[Y1 Y1m Y2 Y2m Y3 Y4]);
      | text(0.5,0.3,'AC6','HorizontalAlignment','center')
      | HaveSPSMec = (strcmp(MechanicalLoad,'Torque Tm') || strcmp(MechanicalLoad,'Speed w'));
      | color('blue');
      | if (HaveSPSMec==1 && strcmp(outputBusMode,'Multiple output buses'))
      |     port_label('input',2,INp)
      |     port_label('output',4,OUTp)
      | end
      | if (HaveSPSMec==1 && strcmp(outputBusMode,'Single output bus'))
      |     port_label('input',2,INp)
      |     port_label('output',2,OUTp)
      | end
  PM Synchronous Motor Drive1 : electricdrivelib/AC drives/PM Synchronous Motor Drive  Commented=on  Rs=0.2  Lls=8.5e-3  Lms=8.5e-3  MachineConstant=Flux linkage established by magnets (V.s)  FluxCst=0.175  VoltageCst=126.966  TorqueCst=1.05  ia=0  ib=0  J=0.089  Friction=0.005  p=4  wm=0  thetam=0  Rsnb_rec=10e3  Csnb_rec=20e-9  Ron_rec=1e-3  Vf_rec=1.3  cap_bus=2000e-6  Rbrake=8  fbrake=4000  activationVoltage=320  shutdownVoltage=310  sourceFrequency=60  deviceType=IGBT / Diodes  Ron_inv=1e-3  Vf_inv=0.8  Vfd_inv=0.8  Tf=1e-6  Tt=2e-6  Tf_GTO=0  Tt_GTO=0  Rsnb_inv=5000  Csnb_inv=inf  regulationType=Speed regulation  Acc=1000  Dec=-1000  kp_sc=5  ki_sc=100  fc_sc=100  Tsc=7*20e-6  Tmin=-17.8  Tmax=17.8  modulationType=Hysteresis  h=0.1  kp_Id=200  ki_Id=1000  kp_Iq=200  ki_Iq=1000  fc_bus=50  car_freq=20000  freq_max=20e3  Tvect=20e-6  baseSampleTime=2e-06  outputBusMode=Multiple output buses  busLabels=off  MechanicalLoad=Torque Tm  modelDetailLevel=Detailed  driveType=AC6  AverageValue=off
      link override VECT: machineConstant=Flux linkage established by magnets (V.s)
      settings: SourceProductName=Simscape Power Systems  SourceProductBaseCode=PS
  + : PMIOPort  Port=1  Side=Left
  - : PMIOPort  Port=2  Side=Left
  wm : Outport
  Feedback : Outport  Port=2
  wires:
  Speed (rad/sec)/1 -> PM Synchronous Motor Drive/1(SP)
  Trq (Nm)/1 -> PM Synchronous Motor Drive/2(Tm)
  PM Synchronous Motor Drive/3(Ctrl) -> Bus Creator/3
  PM Synchronous Motor Drive/2(Conv.) -> Bus Selector/1, Bus Creator/2
  PM Synchronous Motor Drive/1(Motor) -> Bus Creator/1
  PM Synchronous Motor Drive/4(Wm) -> wm/1
  Bus Creator/1 -> Feedback/1
  Bus Selector/1 -> DC_bus overvoltage protection/1(DC_Bus_Voltage)  "<V bus (V)>"
  connections:
  PM Synchronous Motor Drive/LConn1 -- DC_bus overvoltage protection/LConn1 -- +/RConn1
  PM Synchronous Motor Drive/LConn2 -- DC_bus overvoltage protection/LConn2 -- -/RConn1

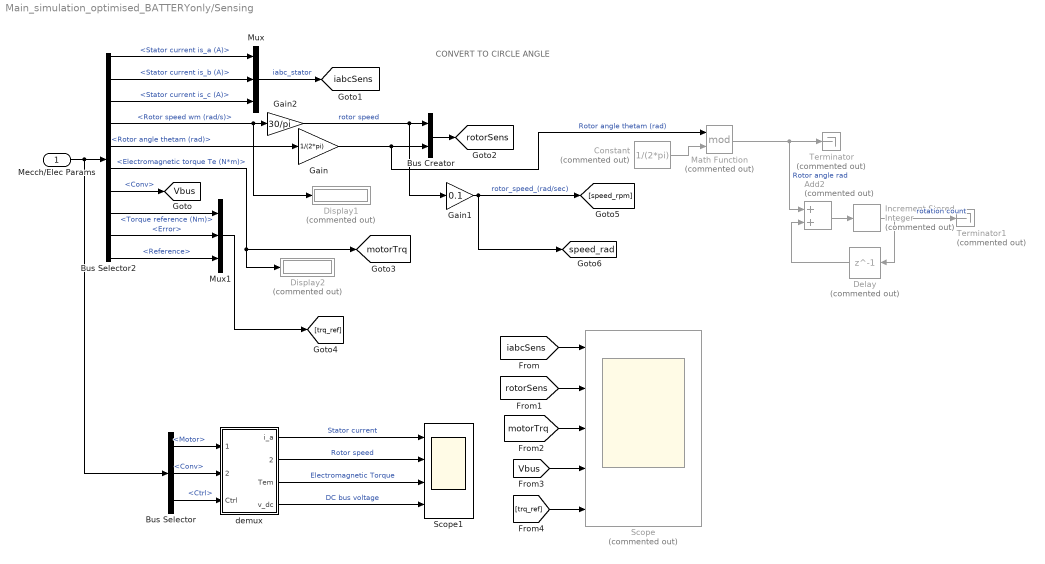
== system Main_simulation_optimised_BATTERYonly/Sensing ==
  note: CONVERT TO CIRCLE ANGLE
  Mecch/Elec Params : Inport
  Add2 : Sum  Commented=on
  Bus Creator : BusCreator  Inputs=2
  Bus Selector : BusSelector  OutputSignals=Motor,Conv,Ctrl
  Bus Selector2 : BusSelector  OutputSignals=Motor.Stator current is_a (A),Motor.Stator current is_b (A),Motor.Stator current is_c (A),Motor.Rotor speed wm (rad/s),Motor.Rotor angle thetam (rad),Motor.Electromagnetic torque Te (N*m),Conv,Ctrl.Torque reference (Nm),Ctrl.Error,Ctrl.Reference
  Constant : Constant  Commented=on  Value=1/(2*pi)
  Delay : Delay  Commented=on  DelayLength=1
  Display1 : Display  Commented=on
  Display2 : Display  Commented=on
  Gain : Gain  Gain=1/(2*pi)
  Gain1 : Gain  Gain=0.1
  Gain2 : Gain  Gain=30/pi  SaturateOnIntegerOverflow=on  OutDataTypeStr=Inherit: Same as input  ParamDataTypeStr=Inherit: Same as input
  Increment Stored Integer : simulink/Additional Math & Discrete/Additional Math: Increment - Decrement/Increment Stored Integer  Commented=on
      settings: SourceProductName=Simulink
  Math Function : Math  Commented=on  Operator=mod  SaturateOnIntegerOverflow=on
  Mux : Mux  Inputs=3
  Mux1 : Mux  Inputs=3
  Scope : Scope  Commented=on  NumInputPorts=5
  Scope1 : Scope  NumInputPorts=4
  Terminator : Terminator  Commented=on
  Terminator1 : Terminator  Commented=on
  demux : Subsystem
  tag scope: Vbus=global, iabcSens=global, motorTrq=global, rotorSens=global, speed_rad=global
  wires:
  Bus Selector2/5 -> Gain/1  "<Rotor angle thetam (rad)>"
  Mux/1 -> [iabcSens]  "iabc_stator"
  Bus Selector2/3 -> Mux/3  "<Stator current is_c (A)>"
  Mecch/Elec Params/1 -> Bus Selector/1, Bus Selector2/1
  Bus Creator/1 -> [rotorSens]
  Bus Selector2/4 -> Display1/1, Gain2/1  "<Rotor speed wm (rad/s)>"
  Bus Selector2/1 -> Mux/1  "<Stator current is_a (A)>"
  Bus Selector2/2 -> Mux/2  "<Stator current is_b (A)>"
  Bus Selector2/6 -> [motorTrq], Display2/1  "<Electromagnetic torque Te (N*m)>"
  Gain/1 -> Math Function/1, Bus Creator/2  "Rotor angle thetam (rad)"
  Bus Selector2/7 -> [Vbus]  "<Conv>"
  Bus Selector2/8 -> Mux1/1  "<Torque reference (Nm)>"
  Bus Selector2/9 -> Mux1/2  "<Error>"
  Bus Selector2/10 -> Mux1/3  "<Reference>"
  Mux1/1 -> [trq_ref]
  [iabcSens] -> Scope/1
  [rotorSens] -> Scope/2
  [motorTrq] -> Scope/3
  [Vbus] -> Scope/4
  [trq_ref] -> Scope/5
  Gain1/1 -> [speed_rad], [speed_rpm]  "rotor_speed_(rad/sec)"
  demux/2(speed) -> Scope1/2  "Rotor speed"
  demux/1(i_a) -> Scope1/1  "Stator current"
  Bus Selector/1 -> demux/1(motor)  "<Motor>"
  Bus Selector/2 -> demux/2(Conv.)  "<Conv>"
  demux/4(v_dc) -> Scope1/4  "DC bus voltage"
  demux/3(Tem) -> Scope1/3  "Electromagnetic Torque"
  Bus Selector/3 -> demux/3(Ctrl)  "<Ctrl>"
  Gain2/1 -> Gain1/1, Bus Creator/1  "rotor speed"
  Math Function/1 -> Add2/1, Terminator/1  "Rotor angle rad"
  Constant/1 -> Math Function/2
  Increment Stored Integer/1 -> Terminator1/1, Delay/1  "rotation count"
  Delay/1 -> Add2/2
  Add2/1 -> Increment Stored Integer/1

== system Main_simulation_optimised_BATTERYonly/Speed and Cooling  ==
  note: -exp(0.1*v/10)
  note: to generate speed based cooling rate
  note: not consiidering drag to keep it linear
  note: Y (kmph) = X(r/s) * 100 (kmph) / 400 (r/s)
  Gain1 : Gain  Gain=0.1/10
  Gain2 : Gain  Gain=100/400
  Math Function : Math  SaturateOnIntegerOverflow=on
  cooling_rate : Gain  Gain=-1
  tag scope: cooling_rate=global
  wires:
  Math Function/1 -> cooling_rate/1
  Gain1/1 -> Math Function/1
  [speed_rad] -> Gain2/1
  Gain2/1 -> Gain1/1
  cooling_rate/1 -> [cooling_rate]

== system Main_simulation_optimised_BATTERYonly/Speed ref2 ==
  Demux : Demux  Tag=STV Demux  Outputs=1
  FromWs : FromWorkspace  Tag=STV FromWs  VariableName=tuvar  SampleTime=0
      SigBuilderData=|
      | common.afterFinalStr = 'Extrapolate'
      | common.sampleTime = 0
      | dataSet.timeRange = [0 20]
      | dataSet.name = 'Group 1'
      | sbobj.Groups.Name = 'Group 1'
      | sbobj.Groups.Signals.Name = 'v_ref'
      | sbobj.Groups.Signals.XData = [0 1 1 2 2 2.39 2.39 3.81 5 5 6.45 6.48 6.8 7 8 8.05 9 9.1 10.2 11.4 11.58 12.5 13 13.46 14 14.26 14.48 15.04 15.2 15.4 15.5 15.64 17 18.1 18.42 18.74 19.3 19.52 20]
      | sbobj.Groups.Signals.YData = [0 5.1 0.2 11 7.5 2.4 0.6 7.1 1.2 0.4 8.7 8.1 15.3 13.2 12.9 11.3 7.1 2 2 9.26428571429 8.9 11.2014285714 16.7 17.2 10.45 11.9709897611 14.3 13.8 9.8 11.95 11.2641638225 12.65 12.65 6.4 0 0 1.3 0 0]
      | sbobj.Groups.TimeRange = [0 20]
  v_ref : Outport  Tag=STV Outport
  wires:
  FromWs/1 -> Demux/1
  Demux/1 -> v_ref/1

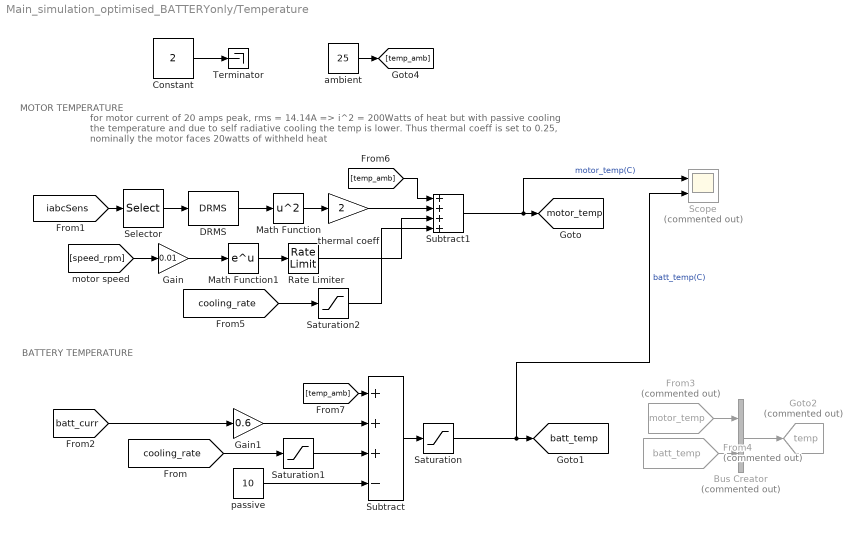
== system Main_simulation_optimised_BATTERYonly/Temperature ==
  note: MOTOR TEMPERATURE
  note: BATTERY TEMPERATURE
  note: for motor current of 20 amps peak, rms = 14.14A => i^2 = 200Watts of heat
      |  but with passive cooling the temperature and due to self radiative cooling the
      | temp is lower. Thus thermal coeff is set to 0.25, nominally the motor faces 20watts of withheld heat
  Bus Creator : BusCreator  Commented=on  Inputs=2
  Constant : Constant  Value=2
  DRMS : sdolib/RMS Blocks/DRMS  Ts=1e-6
      settings: SourceProductName=Simulink Design Optimization  SourceProductBaseCode=SO
  From3 : From  Commented=on  GotoTag=motor_temp  TagVisibility=global
  From4 : From  Commented=on  GotoTag=batt_temp  TagVisibility=global
  Gain : Gain  Gain=0.01
  Gain1 : Gain  Gain=0.6
  Goto2 : Goto  Commented=on  GotoTag=temp  TagVisibility=global
  Math Function : Math  Operator=square  SaturateOnIntegerOverflow=on
  Math Function1 : Math  SaturateOnIntegerOverflow=on
  Rate Limiter : RateLimiter  SampleTimeMode=inherited
  Saturation : Saturate  UpperLimit=48  LowerLimit=20
  Saturation1 : Saturate  UpperLimit=0  LowerLimit=-20
  Saturation2 : Saturate  UpperLimit=0  LowerLimit=-10
  Scope : Scope  Commented=on  NumInputPorts=2
  Selector : Selector  InputPortWidth=3  IndexOptions=Index vector (dialog)  Indices=[1]  OutputSizes=1
  Subtract : Sum  Inputs=+++-
  Subtract1 : Sum  Inputs=++++
  Terminator : Terminator
  ambient : Constant  Value=25
  passive : Constant  Value=10
  thermal coeff : Gain  Gain=2
  tag scope: batt_temp=global, motor_temp=global
  wires:
  Math Function/1 -> thermal coeff/1
  Subtract/1 -> Saturation/1
  passive/1 -> Subtract/4
  Saturation1/1 -> Subtract/3
  [cooling_rate] -> Saturation1/1
  [iabcSens] -> Selector/1
  DRMS/1 -> Math Function/1
  Selector/1 -> DRMS/1
  Saturation/1 -> [batt_temp], Scope/2  "batt_temp(C)"
  thermal coeff/1 -> Subtract1/2
  [speed_rpm] -> Gain/1
  Math Function1/1 -> Rate Limiter/1
  Subtract1/1 -> [motor_temp], Scope/1  "motor_temp(C)"
  Gain/1 -> Math Function1/1
  Rate Limiter/1 -> Subtract1/3
  [batt_curr] -> Gain1/1
  Gain1/1 -> Subtract/2
  From3/1 -> Bus Creator/1
  From4/1 -> Bus Creator/2
  Bus Creator/1 -> Goto2/1
  [cooling_rate] -> Saturation2/1
  Saturation2/1 -> Subtract1/4
  Constant/1 -> Terminator/1
  ambient/1 -> [temp_amb]
  [temp_amb] -> Subtract1/1
  [temp_amb] -> Subtract/1

== system Main_simulation_optimised_BATTERYonly/Torque Ref ==
  Demux : Demux  Tag=STV Demux  Outputs=1
  FromWs : FromWorkspace  Tag=STV FromWs  VariableName=tuvar  SampleTime=0
      SigBuilderData=|
      | common.afterFinalStr = 'Extrapolate'
      | common.sampleTime = 0
      | dataSet.timeRange = [0 20]
      | dataSet.name = 'Group 1'
      | sbobj.Groups.Name = 'Group 1'
      | sbobj.Groups.Signals.Name = 'Signal 2'
      | sbobj.Groups.Signals.XData = [0 1 1.3 2 2 2.39 2.39 3.81 4.29 4.6 6.1 6.45 6.55 6.55 8 9 9.4 10 20]
      | sbobj.Groups.Signals.YData = [2.05 9.95 -8.5 13.8 -5 6.5 -5.2 7 -8.4 -1.3 8.7 -4.1 14.7 -1.9 11.6 11.5 -5.3 0 0]
      | sbobj.Groups.TimeRange = [0 20]
  Signal 2 : Outport  Tag=STV Outport
  wires:
  Demux/1 -> Signal 2/1
  FromWs/1 -> Demux/1

== system Main_simulation_optimised_BATTERYonly/Velocity_profile selector ==
  Bus Creator : BusCreator  Inputs=5
  Bus Selector : BusSelector  OutputSignals=Jap10 (135s)
  Drive Cycle Source : autolibshared/Drive Cycle Source  cycleVar=IM240  tfinal="240  seconds"  cycleRepeat=off  outAccPort=off  t_wot1=5  xdot_woto=0  xdot_wot1=30  t_wot2=20  xdot_wot2=0  t_wotend=30  srcUnit=m/s  outUnit=m/s  srcAccUnit=m/s/s  outAccUnit=m/s^2  dt=100e-6
      settings: SourceProductName=Powertrain Blockset  SourceProductBaseCode=PW
  Drive Cycle Source1 : autolibshared/Drive Cycle Source  cycleVar=NYCC  tfinal="598  seconds"  cycleRepeat=off  outAccPort=off  t_wot1=5  xdot_woto=0  xdot_wot1=30  t_wot2=20  xdot_wot2=0  t_wotend=30  srcUnit=m/s  outUnit=m/s  srcAccUnit=m/s/s  outAccUnit=m/s^2  dt=100e-6
      settings: SourceProductName=Powertrain Blockset  SourceProductBaseCode=PW
  Drive Cycle Source2 : autolibshared/Drive Cycle Source  cycleVar=FTP75  tfinal="2474  seconds"  cycleRepeat=off  outAccPort=off  t_wot1=5  xdot_woto=0  xdot_wot1=30  t_wot2=20  xdot_wot2=0  t_wotend=30  srcUnit=m/s  outUnit=m/s  srcAccUnit=m/s/s  outAccUnit=m/s^2  dt=100e-6
      settings: SourceProductName=Powertrain Blockset  SourceProductBaseCode=PW
  Drive Cycle Source3 : autolibshared/Drive Cycle Source  cycleVar=FTP75  tfinal="2474  seconds"  cycleRepeat=off  outAccPort=off  t_wot1=5  xdot_woto=0  xdot_wot1=30  t_wot2=20  xdot_wot2=0  t_wotend=30  srcUnit=m/s  outUnit=m/s  srcAccUnit=m/s/s  outAccUnit=m/s^2  dt=100e-6
      settings: SourceProductName=Powertrain Blockset  SourceProductBaseCode=PW
  Drive Cycle Source4 : autolibshared/Drive Cycle Source  cycleVar=Japanese 10 Mode  tfinal="135  seconds"  cycleRepeat=off  outAccPort=off  t_wot1=5  xdot_woto=0  xdot_wot1=30  t_wot2=20  xdot_wot2=0  t_wotend=30  srcUnit=m/s  outUnit=m/s  srcAccUnit=m/s/s  outAccUnit=m/s^2  dt=100e-6
      settings: SourceProductName=Powertrain Blockset  SourceProductBaseCode=PW
  Gain : Gain
  Rate Transition : RateTransition
  Vel_reference_user : Outport
  wires:
  Rate Transition/1 -> Vel_reference_user/1  "Vel_reference_user"
  Drive Cycle Source/1 -> Bus Creator/5  "IM240 (240s)"
  Gain/1 -> Rate Transition/1
  Bus Selector/1 -> Gain/1  "<Jap10 (135s)>"
  Drive Cycle Source1/1 -> Bus Creator/3  "NYCC (598s)"
  Drive Cycle Source2/1 -> Bus Creator/4  "CUEDC SPC240 (240s)"
  Bus Creator/1 -> Bus Selector/1
  Drive Cycle Source4/1 -> Bus Creator/1  "Jap10 (135s)"
  Drive Cycle Source3/1 -> Bus Creator/2  "BAC-Arterial Cycle (270s)"

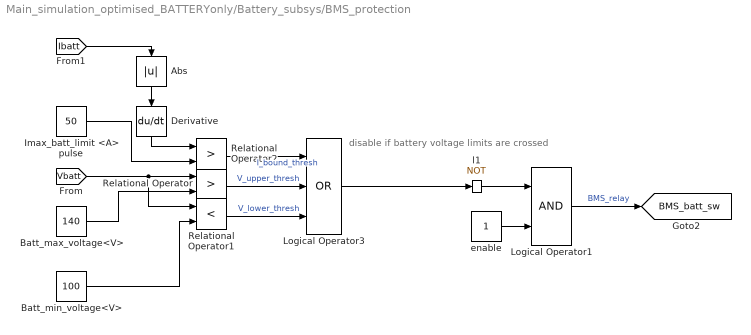
== system Main_simulation_optimised_BATTERYonly/Battery_subsys/BMS_protection ==
  note: disable if battery voltage limits are crossed
  Abs : Abs
  Batt_max_voltage<V> : Constant  Value=140
  Batt_min_voltage<V> : Constant  Value=100
  Derivative : Derivative
  Imax_batt_limit <A> pulse : Constant  Value=50
  Logical Operator1 : Logic  AllPortsSameDT=off  OutDataTypeStr=boolean
  Logical Operator3 : Logic  Operator=OR  Inputs=3  AllPortsSameDT=off  OutDataTypeStr=boolean
  Relational Operator : RelationalOperator  Operator=>  OutDataTypeStr=boolean  RndMeth=Simplest
  Relational Operator1 : RelationalOperator  Operator=<  OutDataTypeStr=boolean  RndMeth=Simplest
  Relational Operator2 : RelationalOperator  Operator=>  OutDataTypeStr=boolean  RndMeth=Simplest
  enable : Constant
  l1 : Logic  Operator=NOT  IconShape=distinctive  AllPortsSameDT=off  OutDataTypeStr=boolean
  tag scope: BMS_batt_sw=global
  wires:
  [Vbatt] -> Relational Operator1/1, Relational Operator/1
  Relational Operator2/1 -> Logical Operator3/1  "I_bound_thresh"
  Imax_batt_limit <A> pulse/1 -> Relational Operator2/2
  [Ibatt] -> Abs/1
  Batt_min_voltage<V>/1 -> Relational Operator1/2
  Logical Operator1/1 -> [BMS_batt_sw]  "BMS_relay"
  Relational Operator/1 -> Logical Operator3/2  "V_upper_thresh"
  l1/1 -> Logical Operator1/1
  Relational Operator1/1 -> Logical Operator3/3  "V_lower_thresh"
  Batt_max_voltage<V>/1 -> Relational Operator/2
  Logical Operator3/1 -> l1/1
  enable/1 -> Logical Operator1/2
  Abs/1 -> Derivative/1
  Derivative/1 -> Relational Operator2/1

== system Main_simulation_optimised_BATTERYonly/Battery_subsys/BMS_relay ==
  Ideal Switch : powerlib/Power Electronics/Ideal Switch  Ron=0.001  Lon=0  IC=1  Rs=1e4  Cs=1e-8  Measurements=off
  Ideal Switch1 : powerlib/Power Electronics/Ideal Switch  Ron=0.001  Lon=0  IC=1  Rs=1e4  Cs=1e-8  Measurements=off
  L : powerlib/Elements/Series RLC Branch  Commented=on  LConnTagsString=__new0  RConnTagsString=__new0  BranchType=RL  Resistance=0.001  Inductance=20e-6  SetiL0=off  InitialCurrent=0  Capacitance=10e-6  Setx0=off  InitialVoltage=0  Measurements=None
  +Vo : PMIOPort  Port=1  Side=Right
  +B : PMIOPort  Port=2  Side=Left
  -Vo : PMIOPort  Port=3  Side=Right
  -B : PMIOPort  Port=4  Side=Left
  wires:
  [BMS_batt_sw] -> Ideal Switch/1, Ideal Switch1/1
  connections:
  Ideal Switch1/RConn1 -- -Vo/RConn1
  Ideal Switch1/LConn1 -- -B/RConn1
  Ideal Switch/LConn1 -- +B/RConn1
  +Vo/RConn1 -- Ideal Switch/RConn1
